simulink model "BLDCmotorDerating_R2017b"  (R2017b)
settings: Solver=FixedStepDiscrete  StartTime=0.0  StopTime=15  FixedStep=Ts_ctrl  RelTol=1e-3
values from neighbouring files (symbols this model uses):
  DC_CUR_LIM_CONT = 15    [init_model_derating.m]
  DC_CUR_LIM_PEAK = 20    [init_model_derating.m]
  dt_curLimDer = PWM_LIM_MAX / t_DC_CUR_DER / (f_ctrl / 1000)    (= 0.03)    [init_model_derating.m]
  dt_curLimRec = - PWM_LIM_MAX / t_DC_CUR_REC / (f_ctrl / 1000)    (= -0.03)    [init_model_derating.m]
  f_ctrl = 1/Ts_ctrl    (= 16666.6666667)    [init_model.m]    (also in init_model_derating.m)
libraries: simulink x2, BLDC_controller_Lib x1
settings Model: Creator=eferu  LastModifiedBy=eferu

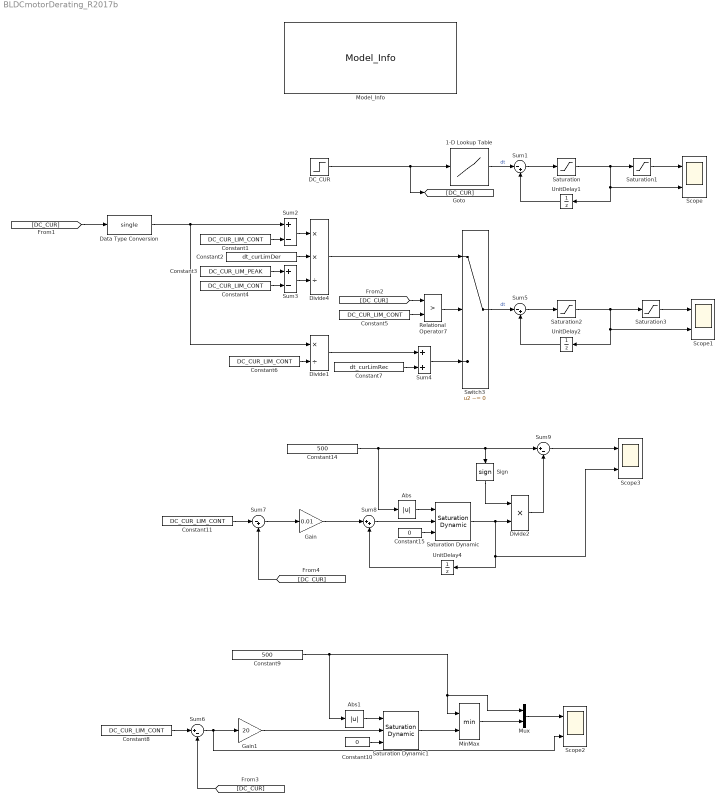
== system BLDCmotorDerating_R2017b ==
  1-D Lookup Table : Lookup_n-D  NumberOfTableDimensions=1  BreakpointsForDimension1=[0 15 20]  Table=[-1000/2 0 1000/2]/f_ctrl  InternalRulePriority=Speed  RndMeth=Simplest  InputSameDT=on
  Abs : Abs
  Abs1 : Abs
  Constant{1,4..6,8,11} (6 alike) : Constant  Value=DC_CUR_LIM_CONT  OutDataTypeStr=Inherit: Inherit via back propagation
  Constant10 : Constant  Value=0  OutDataTypeStr=Inherit: Inherit via back propagation
  Constant14 : Constant  Value=500  OutDataTypeStr=Inherit: Inherit via back propagation
  Constant15 : Constant  Value=0  OutDataTypeStr=Inherit: Inherit via back propagation
  Constant2 : Constant  Value=dt_curLimDer  OutDataTypeStr=Inherit: Inherit via back propagation
  Constant3 : Constant  Value=DC_CUR_LIM_PEAK  OutDataTypeStr=Inherit: Inherit via back propagation
  Constant7 : Constant  Value=dt_curLimRec  OutDataTypeStr=Inherit: Inherit via back propagation
  Constant9 : Constant  Value=500  OutDataTypeStr=Inherit: Inherit via back propagation
  DC_CUR : Step  Time=5  Before=20  After=13  SampleTime=0
  Data Type Conversion : DataTypeConversion  OutDataTypeStr=single
  Divide1 : Product  Inputs=*/  OutDataTypeStr=Inherit: Inherit via back propagation  RndMeth=Simplest
  Divide2 : Product  Inputs=**  OutDataTypeStr=Inherit: Inherit via back propagation  RndMeth=Simplest
  Divide4 : Product  Inputs=**/  OutDataTypeStr=Inherit: Inherit via back propagation  RndMeth=Simplest
  Gain : Gain  Tag=struct('comment',struct('text','','placement',1),'logdata',struct('maxnumvals',inf,'plotchannels',[],'loggingmode',3,'channels',1),'output',struct('variable','','description','','name','$S_$B','width',1,'address','','max',NaN,'min',NaN,'class','default','type','CONTINUOUS','scaling','','lsb',1,'offset',0,'arb',0,'freeze',1,'unit','','autoscalingmode',1,'lowerheadroom',1,'upperheadroom',1,'headroomunit','bit','keepdatatype',1,'checkmin',0,'checkmax',0,'castoutput',0,'show',0),'gain',struct('variable','','description','','name','$S_$B_gain','width',1,'address','','max',NaN,'min',NaN,'class','default','type','CONTINUOUS','scaling','','lsb',1,'offset',0,'arb',0,'freeze',1,'unit','','keepdatatype',1,'value','1','scalar',0,'tolerance',1),'scalingvalid',0,'date',730486)  Gain=0.01  RndMeth=Zero  SaturateOnIntegerOverflow=on  OutDataTypeStr=Inherit: Same as input  ParamDataTypeStr=Inherit: Same as input
  Gain1 : Gain  Tag=struct('comment',struct('text','','placement',1),'logdata',struct('maxnumvals',inf,'plotchannels',[],'loggingmode',3,'channels',1),'output',struct('variable','','description','','name','$S_$B','width',1,'address','','max',NaN,'min',NaN,'class','default','type','CONTINUOUS','scaling','','lsb',1,'offset',0,'arb',0,'freeze',1,'unit','','autoscalingmode',1,'lowerheadroom',1,'upperheadroom',1,'headroomunit','bit','keepdatatype',1,'checkmin',0,'checkmax',0,'castoutput',0,'show',0),'gain',struct('variable','','description','','name','$S_$B_gain','width',1,'address','','max',NaN,'min',NaN,'class','default','type','CONTINUOUS','scaling','','lsb',1,'offset',0,'arb',0,'freeze',1,'unit','','keepdatatype',1,'value','1','scalar',0,'tolerance',1),'scalingvalid',0,'date',730486)  Gain=20  RndMeth=Zero  SaturateOnIntegerOverflow=on  OutDataTypeStr=Inherit: Same as input  ParamDataTypeStr=Inherit: Same as input
  MinMax : MinMax  Inputs=2
  Model_Info : BLDC_controller_Lib/Model_Info
  Mux : Mux  Inputs=2
  Relational Operator7 : RelationalOperator  Operator=>  OutDataTypeStr=boolean  RndMeth=Simplest
  Saturation : Saturate  UpperLimit=1000  LowerLimit=-inf
  Saturation Dynamic : simulink/Discontinuities/Saturation Dynamic  OutMin=[]  OutMax=[]  OutDataTypeStr=Inherit: Same as second input  OutDataType=fixdt(1, 16)  OutScaling=2^-10  DoSatur=off
  Saturation Dynamic1 : simulink/Discontinuities/Saturation Dynamic  OutMin=[]  OutMax=[]  OutDataTypeStr=Inherit: Same as second input  OutDataType=fixdt(1, 16)  OutScaling=2^-10  DoSatur=off
  Saturation1 : Saturate  UpperLimit=1000  LowerLimit=0
  Saturation2 : Saturate  UpperLimit=1000*100  LowerLimit=-60000  RndMeth=Simplest
  Saturation3 : Saturate  UpperLimit=1000  LowerLimit=0
  Scope{,1..3} (4 alike) : Scope  NumInputPorts=2
  Sign : Signum
  Sum1 : Sum  Inputs=|-+  RndMeth=Simplest  InputSameDT=on  OutDataTypeStr=Inherit: Same as first input
  Sum2 : Sum  Inputs=+-  RndMeth=Simplest  InputSameDT=on  OutDataTypeStr=Inherit: Same as first input
  Sum3 : Sum  Inputs=+-  RndMeth=Simplest  InputSameDT=on  OutDataTypeStr=Inherit: Same as first input
  Sum4 : Sum  RndMeth=Simplest  InputSameDT=on  OutDataTypeStr=Inherit: Same as first input
  Sum5 : Sum  Inputs=|-+  RndMeth=Simplest  InputSameDT=on  OutDataTypeStr=Inherit: Same as first input
  Sum6 : Sum  Inputs=|+-  RndMeth=Simplest  InputSameDT=on  OutDataTypeStr=Inherit: Same as first input
  Sum7 : Sum  Inputs=|-+  RndMeth=Simplest  InputSameDT=on  OutDataTypeStr=Inherit: Same as first input
  Sum8 : Sum  Inputs=|++  RndMeth=Simplest  InputSameDT=on  OutDataTypeStr=Inherit: Same as first input
  Sum9 : Sum  Inputs=|+-  RndMeth=Simplest  InputSameDT=on  OutDataTypeStr=Inherit: Same as first input
  Switch3 : Switch  Criteria=u2 ~= 0  OutDataTypeStr=Inherit: Inherit via back propagation  RndMeth=Zero
  UnitDelay1 : UnitDelay  InitialCondition=1000  SampleTime=-1
  UnitDelay2 : UnitDelay  InitialCondition=1000  SampleTime=-1
  UnitDelay4 : UnitDelay  SampleTime=-1
  wires:
  UnitDelay1/1 -> Sum1/2
  DC_CUR/1 -> [DC_CUR], 1-D Lookup Table/1
  1-D Lookup Table/1 -> Sum1/1  "dt"
  Sum1/1 -> Saturation/1
  Saturation1/1 -> Scope/1
  Saturation/1 -> Saturation1/1, Scope/2, UnitDelay1/1
  Constant5/1 -> Relational Operator7/2
  Relational Operator7/1 -> Switch3/2
  Constant1/1 -> Sum2/2
  Sum2/1 -> Divide4/1
  Constant2/1 -> Divide4/2
  Sum3/1 -> Divide4/3
  Constant3/1 -> Sum3/1
  Constant4/1 -> Sum3/2
  Divide4/1 -> Switch3/1
  [DC_CUR] -> Relational Operator7/1
  [DC_CUR] -> Data Type Conversion/1
  Divide1/1 -> Sum4/1
  Sum4/1 -> Switch3/3
  Saturation3/1 -> Scope1/1
  Sum5/1 -> Saturation2/1
  Switch3/1 -> Sum5/1  "dt"
  UnitDelay2/1 -> Sum5/2
  Constant6/1 -> Divide1/2
  Constant7/1 -> Sum4/2
  Data Type Conversion/1 -> Divide1/1, Sum2/1
  Saturation2/1 -> Saturation3/1, UnitDelay2/1, Scope1/2
  UnitDelay4/1 -> Sum8/2
  Divide2/1 -> Sum9/2
  Constant11/1 -> Sum7/1
  [DC_CUR] -> Sum7/2
  Sum8/1 -> Saturation Dynamic/2
  Constant15/1 -> Saturation Dynamic/3
  Sum7/1 -> Gain/1
  Sum9/1 -> Scope3/1
  Gain/1 -> Sum8/1
  Saturation Dynamic/1 -> Scope3/2, UnitDelay4/1, Divide2/2
  Sign/1 -> Divide2/1
  Abs/1 -> Saturation Dynamic/1
  Constant14/1 -> Abs/1, Sum9/1, Sign/1
  Sum6/1 -> Scope2/2, Gain1/1
  [DC_CUR] -> Sum6/2
  Constant8/1 -> Sum6/1
  MinMax/1 -> Mux/2
  Mux/1 -> Scope2/1
  Constant9/1 -> Abs1/1, MinMax/1, Mux/1
  Abs1/1 -> Saturation Dynamic1/1
  Constant10/1 -> Saturation Dynamic1/3
  Gain1/1 -> Saturation Dynamic1/2
  Saturation Dynamic1/1 -> MinMax/2
